simulink model "Robot3GDL2015"  (R2022a)
settings: Solver=ode45  StartTime=0.0  StopTime=Tfinal  RelTol=1e-3
undefined symbols (not defined in the file or in its folder): Cilindric_mgd, MGI, Tem
settings Model: Creator=Shadow  LastModifiedBy=Shadow
settings SolverCC: AlgebraicLoopSolver=TrustRegion
settings OptimizationCC: LifeSpan=inf
settings DebuggingCC: UnconnectedInputMsg=warning  UnconnectedOutputMsg=warning  UnconnectedLineMsg=warning  SFExecutionAtInitializationDiag=none  SFMachineParentedDataDiag=warning  ArithmeticOperatorsInVariantConditions=warning
settings HardwareCC: ProdBitPerSizeT=32  ProdBitPerPtrDiffT=32  ProdWordSize=32  ProdHWDeviceType=Specified
settings SFSimCC: CustomCodeUndefinedFunction=UseInterfaceOnly
settings CodeAppCC: StateflowObjectComments=on

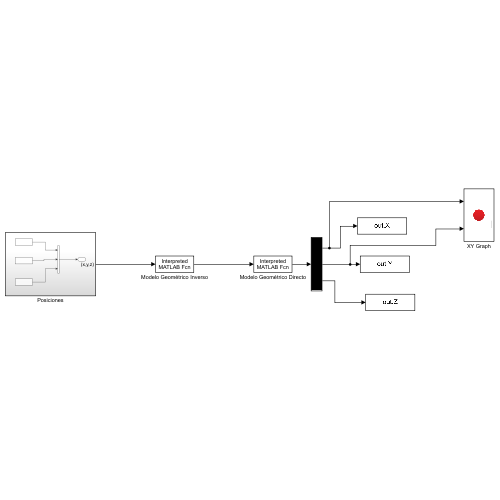
[thumbnail: Simulink's stored preview of the top-level diagram]
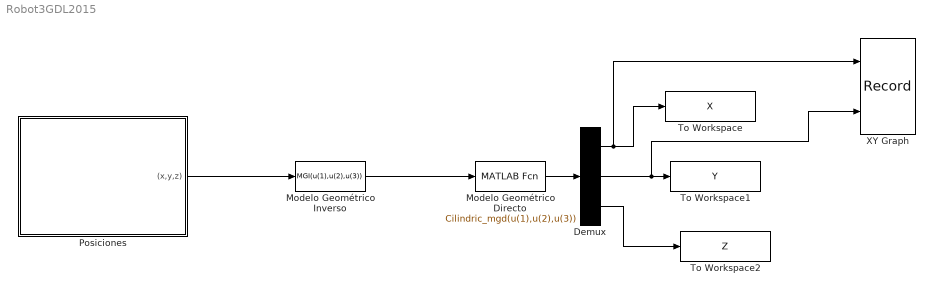
== system Robot3GDL2015 ==
  Demux : Demux  Outputs=3
  Modelo Geométrico Directo : MATLABFcn  MATLABFcn=Cilindric_mgd(u(1),u(2),u(3))  OutputDimensions=3
  Modelo Geométrico Inverso : MATLABFcn  MATLABFcn=MGI(u(1),u(2),u(3))  OutputDimensions=3
  Posiciones : Subsystem
  To Workspace : ToWorkspace  VariableName=X
  To Workspace1 : ToWorkspace  VariableName=Y
  To Workspace2 : ToWorkspace  VariableName=Z
  XY Graph : Record  FileSettingsInternal="{\"entries\":[{\"content\":{\"excelSettings\":{\"content\":{},\"type\":\"Streamout.ExcelSettings\"}},\"type\":\"Streamout.FileSettingStorage\",\"uuid\":\"41500efb-46d4-4989-a014-15aa6d46e0a1\"}],\"packageUris\":[\"http://schema.mathworks.com/mf0/streamout_blocks/R2020a\"],\"version\":\"1.0\"}"  Layout=[1 1]  SignalsInternal="{\"entries\":[{\"content\":{\"signals\":[{\"content\":{\"blockPath\":[\"Robot3GDL2015/XY Graph\"],\"channel\":[],\"dimensions\":[1],\"domain\":\"Robot3GDL2015/XY Graph\",\"lineColor\":\"#a2142f\",\"plots\":[1],\"port\":1,\"sid\":[\"\"],\"signalID\":72,\"signalName\":\"Demux:1\"},\"type\":\"RecordBlkView.Signal\",\"uuid\":\"36855a8a-6583-4a14-8ba9-0d956a6c2985\"},{\"content\":{\"blockPath\":[\"Robot3GDL2015/XY Graph\"],\"channel\":[],\"dimensions\":[1],\"domain\":\"Robot3GDL2015/XY Graph\",\"lineColor\":\"#139fff\",\"plots\":[1],\"port\":2,\"sid\":[\"\"],\"signalID\":76,\"signalName\":\"Demux:2\"},\"type\":\"RecordBlkView.Signal\",\"uuid\":\"5ab9a209-30f6-4af3-83aa-3b00413217f3\"}]},\"type\":\"RecordBlkView.InputSignals\",\"uuid\":\"f9bf6519-cb44-4e7e-8da9-5f31d76f1d3e\"}],\"packageUris\":[\"http://schema.mathworks.com/mf0/streamout_blocks/R2020a\"],\"version\":\"1.0\"}"  VisualizationBindings="{\"xyplotplugin\":{\"info\":[{\"series\":[{\"bindingParametersList\":[{\"parameter\":\"X-Axis\",\"signalID\":72,\"signalName\":\"Demux:1\"},{\"parameter\":\"Y-Axis\",\"signalID\":76,\"signalName\":\"Demux:2\"}],\"seriesID\":49832}],\"subplotID\":1}]}}"  CompatibilityTag=XY  st=-1
  wires:
  Demux/2 -> XY Graph/2, To Workspace1/1
  Demux/3 -> To Workspace2/1
  Modelo Geométrico Directo/1 -> Demux/1
  Modelo Geométrico Inverso/1 -> Modelo Geométrico Directo/1
  Posiciones/1((x,y,z)) -> Modelo Geométrico Inverso/1
  Demux/1 -> To Workspace/1, XY Graph/1

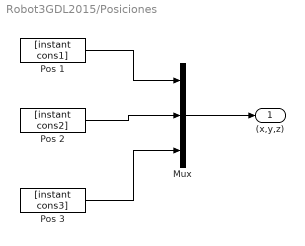
== system Robot3GDL2015/Posiciones ==
  Mux : Mux  Inputs=3
  Pos 1 : FromWorkspace  VariableName=[instant cons1]  SampleTime=Tem  ZeroCross=off
  Pos 2 : FromWorkspace  VariableName=[instant cons2]  SampleTime=Tem  ZeroCross=off
  Pos 3 : FromWorkspace  VariableName=[instant cons3]  SampleTime=Tem  ZeroCross=off
  (x,y,z) : Outport
  wires:
  Pos 3/1 -> Mux/3
  Pos 1/1 -> Mux/1
  Pos 2/1 -> Mux/2
  Mux/1 -> (x,y,z)/1
